simulink subsystem "simscape_model"  (R2024b)
settings: Solver=VariableStepAuto  StartTime=0.0  StopTime=10.0  RelTol=1e-3
libraries: fl_lib x2, nesl_utility x2
settings Model: Creator=eric  LastModifiedBy=eric

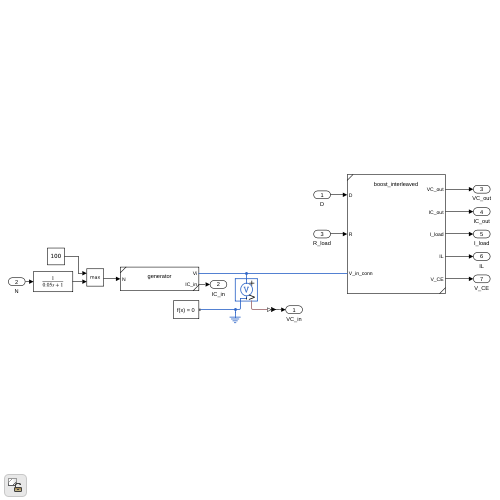
[thumbnail: Simulink's stored preview of the top-level diagram]
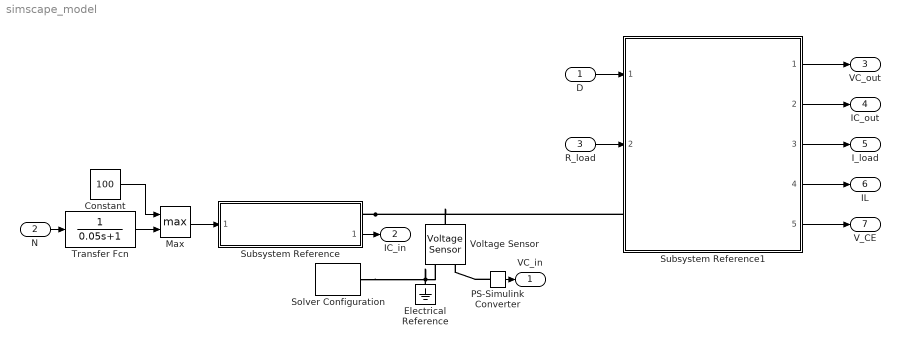
== system simscape_model ==
  D : Inport
  N : Inport  Port=2
  R_load : Inport  Port=3
  Constant : Constant  Value=100
  Electrical Reference : fl_lib/Electrical/Electrical Elements/Electrical Reference
  Max : MinMax  Function=max  Inputs=2
  PS-Simulink Converter : nesl_utility/PS-Simulink Converter  PhysicalDomain=network_engine_domain  SubClassName=ps_output  LeftPortType=input  RightPortType=output  PseudoPeriodic=off  Frequencies=[]  VectorFormat=inherit  Unit=inherit  AffineConversion=off
  Solver Configuration : nesl_utility/Solver Configuration  PhysicalDomain=network_engine_domain  SubClassName=solver  LeftPortType=input  RightPortType=generic  Tones=[]  Harmonics=[]  SimulateNoise=off  Profile=off  UseLocalSampling=off  EnableSwitchedLinearOptims=on  FrequencyDomain=off  UseCCode=off  RelTol=0.001  AbsTol=0.001  MinStep=1e-09  ToWorkspace=off  RevertToSquareIcSolve=off  NumHomotopyIterations=100  PhasorMode=off  PhasorModeNumHarmonics=1  ConsistencySolver=NEWTON_XTOL_AFTER_FTOL  IndexReductionMethod=DerivativeReplacement  DoDC=off  ResidualTolerance=1e-09  ConsistencyTolSource=GLOBAL  ConsistencyAbsTol=0.001  ConsistencyRelTol=0.001  ConsistencyTolFactor=0.001  UseLocalSolver=off  LocalSolverChoice=NE_BACKWARD_EULER_ADVANCER  ResolveIndetEquations=on  FunctionEvalNumThread=1  LocalSolverSampleTime=0.001  DoFixedCost=off  MaxNonlinIter=3  MaxModeIter=2  ComputeImpulses=off  ImpulseIterations=2  LinearAlgebra=auto  LinearAlgebraNumThread=0  EquationFormulation=NE_TIME_EF  DelaysMemoryBudget=1024  AutomaticFiltering=on  FilteringTimeConstant=0.001  PartitionStorageMethod=AS_NEEDED  PartitionMemoryBudget=1024  PartitionMethod=ROBUST  MultibodyUseLocalSolver=off  MultibodyLocalSolverChoice=ODE1  MultibodyLocalSolverSampleTime=0.001
  Subsystem Reference : Subsystem  ReferencedSubsystem=generator
      settings: PortSchema="{\"entries\":[{\"content\":{\"sides\":[{\"content\":{\"connectorIds\":[\"In1\"]},\"type\":\"ConnectorPlacement.EquallySpacedRectSide\",\"uuid\":\"4c68f494-796d-4f0c-8f13-417987bb9088\"},{\"content\":{\"connectorIds\":[\"LConn1\",\"Out1\"],\"side\":\"RIGHT\"},\"type\":\"ConnectorPlacement.EquallySpacedRectSide\",\"uuid\":\"071cd199-76e6-4fb1-9e31-3d46141246ca\"},{\"content\":{\"side\":\"TOP\"},\"type\":\"ConnectorPlacement.EquallySpacedRectSide\",\"uuid\":\"67c2b748-5c83-4b73-adab-e102138b9c72\"}]},\"type\":\"ConnectorPlacement.EquallySpacedConnector\",\"uuid\":\"d4f865f8-cabb-4160-92fa-2fcb4a613789\"}],\"packageUris\":[\"http://schema.mathworks.com/mf0/Connector/R2020b\"],\"version\":\"1.0\"}"
  Subsystem Reference1 : Subsystem  ReferencedSubsystem=boost_interleaved
  Transfer Fcn : TransferFcn  Denominator=[0.05 1]
  Voltage Sensor : fl_lib/Electrical/Electrical Sensors/Voltage Sensor
  VC_in : Outport
  IC_in : Outport  Port=2
  VC_out : Outport  Port=3
  IC_out : Outport  Port=4
  I_load : Outport  Port=5
  IL : Outport  Port=6
  V_CE : Outport  Port=7
  wires:
  PS-Simulink Converter/1 -> VC_in/1
  D/1 -> Subsystem Reference1/1
  R_load/1 -> Subsystem Reference1/2
  Subsystem Reference1/1 -> VC_out/1
  Subsystem Reference1/3 -> I_load/1
  Subsystem Reference/1 -> IC_in/1
  Subsystem Reference1/4 -> IL/1
  Subsystem Reference1/5 -> V_CE/1
  Subsystem Reference1/2 -> IC_out/1
  Max/1 -> Subsystem Reference/1
  Transfer Fcn/1 -> Max/2
  N/1 -> Transfer Fcn/1
  Constant/1 -> Max/1
  connections:
  Electrical Reference/LConn1 -- Voltage Sensor/RConn2 -- Solver Configuration/RConn1
  Subsystem Reference/LConn1 -- Subsystem Reference1/LConn1 -- Voltage Sensor/LConn1
  PS-Simulink Converter/LConn1 -- Voltage Sensor/RConn1
